simulink model "libyjzx"  (R2020a)
settings: Solver=VariableStepAuto  StartTime=0.0  StopTime=86400  RelTol=1e-3
values from neighbouring files (symbols this model uses):
  t12filt = Hd.Numerator ./ sum(Hd.Numerator)    [acMdl.m]
libraries: cstblocks x1
settings Model: Creator=iorioikawa  LastModifiedBy=iorioikawa
settings OptimizationCC: DefaultParameterBehavior=Inlined  UseDivisionForNetSlopeComputation=on  GainParamInheritBuiltInType=on  UseFloatMulNetSlope=on  EnhancedBackFolding=on  PassReuseOutputArgsAs=Individual arguments  ZeroExternalMemoryAtStartup=off  ZeroInternalMemoryAtStartup=off  LifeSpan=365  OptimizeBlockOrder=speed  DifferentSizesBufferReuse=on  OptimizationCustomize=off  EfficientTunableParamExpr=on
settings DebuggingCC: ParameterTunabilityLossMsg=error
settings SFSimCC: MATLABDynamicMemAlloc=off
settings RTWCC: SystemTargetFile=ert.tlc  TemplateMakefile=ert_default_tmf
settings CodeAppCC: ForceParamTrailComments=on  IgnoreCustomStorageClasses=off  OperatorAnnotations=on  SimulinkDataObjDesc=on  SFDataObjDesc=on  InsertBlockDesc=on
settings ERTTargetCC: TargetLangStandard=C99 (ISO)  GenerateSampleERTMain=on  InlinedParameterPlacement=NonHierarchical  ERTCustomFileTemplate=example_file_process.tlc

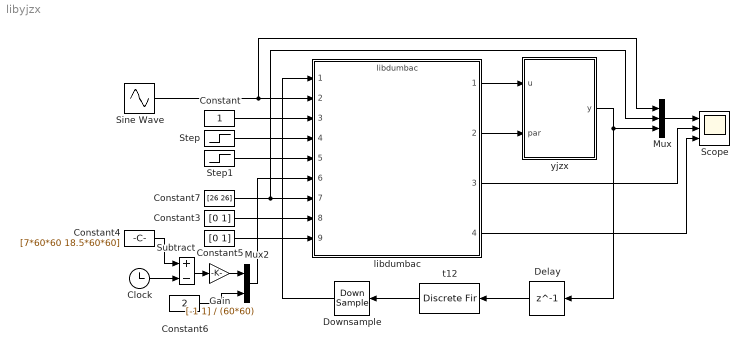
== system libyjzx ==
  Clock : Clock
      settings: Decimation=60*60
  Constant : Constant
  Constant3 : Constant  Value=[0 1]
  Constant4 : Constant  Value=[7*60*60 18.5*60*60]
  Constant5 : Constant  Value=[0 1]
  Constant6 : Constant  Value=2
  Constant7 : Constant  Value=[26 26]
  Delay : Delay  DelayLength=1  InitialCondition=0  SampleTime=1/5
  Downsample : DownSample  N=50
  Gain : Gain  Gain=[-1 1] / (60*60)
  Mux : Mux  Inputs=3
  Mux2 : Mux  Inputs=2
  Scope : Scope  NumInputPorts=3
  Sine Wave : Sin  Amplitude=0.1  Bias=13.26  Frequency=2*pi/24/60/60  Phase=-110/180*pi  SampleTime=0
  Step : Step  Time=3e4  Before=1.5  After=0  SampleTime=0
  Step1 : Step  Time=3e4  Before=1.5  After=3  SampleTime=0
  Subtract : Sum  Inputs=+-
  libdumbac : ModelReference  ModelNameDialog=libdumbac  SimulationMode=Normal  ModelReferenceVersion=1.155
  t12 : DiscreteFir  Coefficients=t12filt
  yjzx : Subsystem
  wires:
  libdumbac/1 -> yjzx/1(u)
  libdumbac/2 -> yjzx/2(par)
  yjzx/1(y) -> Delay/1, Mux/3
  Mux/1 -> Scope/1
  Sine Wave/1 -> Mux/1, libdumbac/2
  Constant/1 -> libdumbac/3
  Step/1 -> libdumbac/4
  Step1/1 -> libdumbac/5
  Constant7/1 -> Mux/2, libdumbac/7
  Constant3/1 -> libdumbac/8
  Constant5/1 -> libdumbac/9
  t12/1 -> Downsample/1
  Delay/1 -> t12/1
  libdumbac/3 -> Scope/2
  Downsample/1 -> libdumbac/1
  libdumbac/4 -> Scope/3
  Clock/1 -> Subtract/2
  Constant4/1 -> Subtract/1
  Subtract/1 -> Gain/1
  Gain/1 -> Mux2/1
  Constant6/1 -> Mux2/2
  Mux2/1 -> libdumbac/6

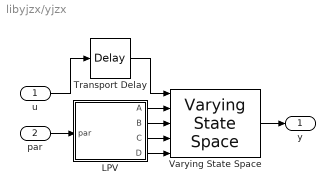
== system libyjzx/yjzx ==
  u : Inport
  par : Inport  Port=2
  LPV : Subsystem
  Transport Delay : TransportDelay  DelayTime=[10 10 0 0 0 0 0 0]
  Varying State Space : cstblocks/Linear Parameter Varying/Varying State Space  x0=[24.665 0 3.78 0]  xNames=''  OutputX=off  OutputDX=off
  y : Outport
  wires:
  LPV/3(C) -> Varying State Space/4
  Varying State Space/1 -> y/1
  LPV/2(B) -> Varying State Space/3
  par/1 -> LPV/1(par)
  u/1 -> Transport Delay/1
  LPV/1(A) -> Varying State Space/2
  LPV/4(D) -> Varying State Space/5
  Transport Delay/1 -> Varying State Space/1

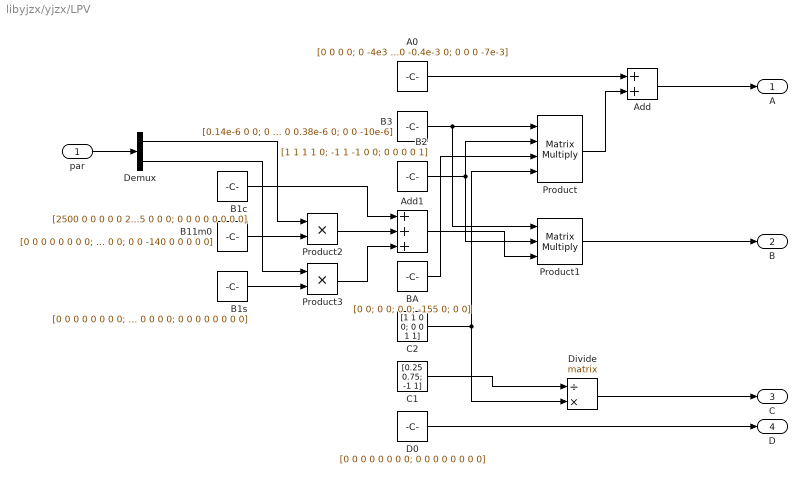
== system libyjzx/yjzx/LPV ==
  par : Inport
  A0 : Constant  Value=[0 0 0 0; 0 -4e3 0 0; 0 0 -0.4e-3 0; 0 0 0 -7e-3]
  Add : Sum
  Add1 : Sum  Inputs=+++
  B11m0 : Constant  Value=[0 0 0 0 0 0 0 0; 0 0 0 0 0 0 0 0; 0 0 -350 0 0 0 0 0; 0 0 0 0 0 0 0 0; 0 0 -140 0 0 0 0 0]
  B1c : Constant  Value=[2500 0 0 0 0 0 200 0; 0 2500 0 0 0 1100 0 300; 0 0 0 -50 0 0 0 0; 0 0 0 0 155 0 0 0; 0 0 0 0 0 0 0 0]
  B1s : Constant  Value=[0 0 0 0 0 0 0 0; 0 0 0 0 0 0 0 0; 0 0 0 1 0 0 0 0; 0 0 0 0 0 0 0 0; 0 0 0 0 0 0 0 0]
  B2 : Constant  Value=[1 1 1 1 0; -1 1 -1 0 0; 0 0 0 0 1]
  B3 : Constant  Value=[0.14e-6 0 0; 0 0 2e-6; 0 0.38e-6 0; 0 0 -10e-6]
  BA : Constant  Value=[0 0; 0 0; 0 0; -155 0; 0 0]
  C1 : Constant  Value=[0.25 0.75; -1 1]
  C2 : Constant  Value=[1 1 0 0; 0 0 1 1]
  D0 : Constant  Value=[0 0 0 0 0 0 0 0; 0 0 0 0 0 0 0 0]
  Demux : Demux  Outputs=2
  Divide : Product  Inputs=/*  Multiplication=Matrix(*)
  Product : Product  Inputs=4  Multiplication=Matrix(*)
  Product1 : Product  Inputs=3  Multiplication=Matrix(*)
  Product2 : Product
  Product3 : Product
  A : Outport
  B : Outport  Port=2
  C : Outport  Port=3
  D : Outport  Port=4
  wires:
  Add1/1 -> Product1/3
  C1/1 -> Divide/1
  Product1/1 -> B/1
  B2/1 -> Product1/2, Product/2
  B1c/1 -> Add1/1
  D0/1 -> D/1
  A0/1 -> Add/1
  Add/1 -> A/1
  Product/1 -> Add/2
  BA/1 -> Product/3
  Divide/1 -> C/1
  C2/1 -> Divide/2, Product/4
  B3/1 -> Product1/1, Product/1
  B11m0/1 -> Product2/2
  Product2/1 -> Add1/2
  Product3/1 -> Add1/3
  B1s/1 -> Product3/2
  par/1 -> Demux/1
  Demux/1 -> Product2/1
  Demux/2 -> Product3/1
